simulink model "acc_hardware"  (R2020a)
settings: Solver=VariableStepAuto  StartTime=0.0  StopTime=inf  RelTol=1e-3
libraries: arduinolib x3, arduinosensorlib x1
settings Model: Creator=shesh  LastModifiedBy=shesh

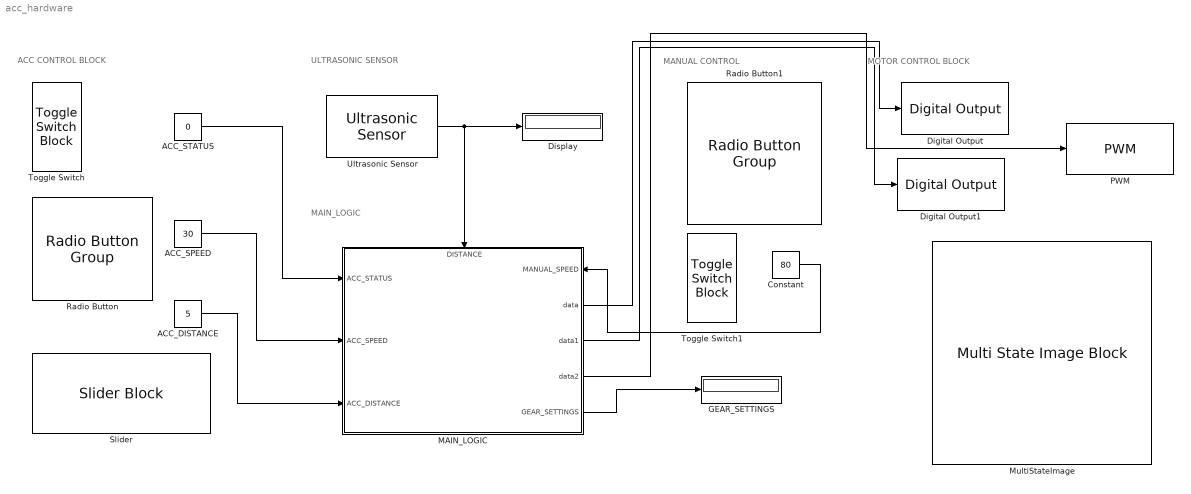
== system acc_hardware ==
  note: MOTOR CONTROL BLOCK
  note: MANUAL CONTROL
  note: MAIN_LOGIC
  note: ULTRASONIC SENSOR
  note: ACC CONTROL BLOCK
  ACC_DISTANCE : Constant  Value=5
  ACC_SPEED : Constant  Value=30
  ACC_STATUS : Constant  Value=0
  Constant : Constant  Value=80
  Digital Output : arduinolib/Digital Output  pinNumber=10  Direction=output  blockPlatform=arduino
  Digital Output1 : arduinolib/Digital Output  pinNumber=9  Direction=output  blockPlatform=arduino
  Display : Display
  GEAR_SETTINGS : Display
  MAIN_LOGIC : Stateflow chart  TreatAsAtomicUnit=on
      settings: PortSchema="{\"entries\":[{\"content\":{\"sides\":[{\"content\":{\"connectorIds\":[\"In3\",\"In4\",\"In5\"]},\"type\":\"ConnectorPlacement.EquallySpacedRectSide\",\"uuid\":\"9577933f-3cd5-4877-b3f1-1cabc5f66bc2\"},{\"content\":{\"connectorIds\":[\"In1\",\"Out1\",\"Out2\",\"Out3\",\"Out4\"],\"side\":\"RIGHT\"},\"type\":\"ConnectorPlacement.EquallySpacedRectSide\",\"uuid\":\"2a6dc85d-fd72-47ef-ac66-14217eaecbf8\"},{\"content\":{\"connectorIds\":[\"In2\"],\"side\":\"TOP\"},\"type\":\"ConnectorPlacement.EquallySpacedRectSide\",\"uuid\":\"38d285f4-ccf6-4804-ae1f-6877806054a5\"}]},\"type\":\"ConnectorPlacement.EquallySpacedConnector\",\"uuid\":\"df4108ed-a8cc-4829-9830-7e09486e0f89\"}],\"packageUris\":[\"http://schema.mathworks.com/mf0/Connector/19700101\"],\"version\":\"1.0\"}"
  MultiStateImage : MultiStateImageBlock
  PWM : arduinolib/PWM  pinNumber=5  frequencyType=Default  desiredFrequency=490.2  achievableFrequency=490.2
  Radio Button : RadioButtonGroup  SelectedLabel=30 KMPH  ButtonGroupName=Group
      settings: Values={{'30 KMPH', '40 KMPH', '50 KMPH', '60 KMPH'}, [30 40 50 60]}
  Radio Button1 : RadioButtonGroup  SelectedLabel=80 KMPH  ButtonGroupName=Group
      settings: Values={{'40 KMPH', '80 KMPH', '120 KMPH', '160 KMPH', 'BREAK'}, [40 80 120 160 0]}
  Slider : SliderBlock  ScaleMin=5  ScaleMax=10  TickInterval=1
  Toggle Switch : ToggleSwitchBlock
      settings: Values={{'Off', 'On'}, [0 1]}
  Toggle Switch1 : ToggleSwitchBlock
      settings: Values={{'Off', 'On'}, [1 0]}
  Ultrasonic Sensor : arduinosensorlib/Ultrasonic Sensor  NumSignalPins=2  TrigPin=4  EchoPin=5  SignalPin=3  SampleTime_=0.1  blockPlatform=ARDUINO
      settings: SourceProductBaseCode=ARDUINO
  wires:
  ACC_STATUS/1 -> MAIN_LOGIC/3(ACC_STATUS)
  ACC_SPEED/1 -> MAIN_LOGIC/4(ACC_SPEED)
  ACC_DISTANCE/1 -> MAIN_LOGIC/5(ACC_DISTANCE)
  MAIN_LOGIC/4(GEAR_SETTINGS) -> GEAR_SETTINGS/1
  Constant/1 -> MAIN_LOGIC/1(MANUAL_SPEED)
  Ultrasonic Sensor/1 -> Display/1, MAIN_LOGIC/2(DISTANCE)
  MAIN_LOGIC/1(data) -> Digital Output/1
  MAIN_LOGIC/2(data1) -> Digital Output1/1
  MAIN_LOGIC/3(data2) -> PWM/1

== stateflow chart acc_hardware/MAIN_LOGIC ==
  state ADAPTIVE_CONTROL_ACTIVE
    entry:
    state ZERO_GEAR_STATE
      entry:
      GEAR_SETTINGS = 0;
    state FRIST_GEAR_STATE
      entry:
      GEAR_SETTINGS = 1;
    state SECOND_GEAR_STATE
      entry:
      GEAR_SETTINGS = 2;
    state BREAKING_STATE
      entry:
      GEAR_SETTINGS = 3;
    (default) -> ADAPTIVE_CONTROL_ACTIVE.ZERO_GEAR_STATE
    ADAPTIVE_CONTROL_ACTIVE.FRIST_GEAR_STATE -> ADAPTIVE_CONTROL_ACTIVE.ZERO_GEAR_STATE : [ACC_SPEED<=40]
    ADAPTIVE_CONTROL_ACTIVE.ZERO_GEAR_STATE -> ADAPTIVE_CONTROL_ACTIVE.FRIST_GEAR_STATE
    ADAPTIVE_CONTROL_ACTIVE.SECOND_GEAR_STATE -> ADAPTIVE_CONTROL_ACTIVE.ZERO_GEAR_STATE : [ACC_SPEED<=40]
    ADAPTIVE_CONTROL_ACTIVE.BREAKING_STATE -> ADAPTIVE_CONTROL_ACTIVE.ZERO_GEAR_STATE : [ACC_SPEED<=40]
  state ADAPTIVE_CONTROL_INACTIVE
    entry:
    state ZERO_GEAR_STATE
      entry:
      GEAR_SETTINGS = 0;
    state FRIST_GEAR_STATE
      entry:
      GEAR_SETTINGS = 1;
    state SECOND_GEAR_STATE
      entry:
      GEAR_SETTINGS = 2;
    state BREAKING_STATE
      entry:
      GEAR_SETTINGS = 3;
    ADAPTIVE_CONTROL_INACTIVE.ZERO_GEAR_STATE -> ADAPTIVE_CONTROL_INACTIVE.FRIST_GEAR_STATE [order 1] : [MANUAL_SPEED == 120]
    ADAPTIVE_CONTROL_INACTIVE.FRIST_GEAR_STATE -> ADAPTIVE_CONTROL_INACTIVE.ZERO_GEAR_STATE [order 3] : [(MANUAL_SPEED == 40) || (MANUAL_SPEED == 80)]
    (default) -> ADAPTIVE_CONTROL_INACTIVE.ZERO_GEAR_STATE
    ADAPTIVE_CONTROL_INACTIVE.ZERO_GEAR_STATE -> ADAPTIVE_CONTROL_INACTIVE.BREAKING_STATE [order 3] : [MANUAL_SPEED == 160]
    ADAPTIVE_CONTROL_INACTIVE.SECOND_GEAR_STATE -> ADAPTIVE_CONTROL_INACTIVE.FRIST_GEAR_STATE [order 1] : [MANUAL_SPEED == 120]
    ADAPTIVE_CONTROL_INACTIVE.SECOND_GEAR_STATE -> ADAPTIVE_CONTROL_INACTIVE.ZERO_GEAR_STATE [order 3] : [(MANUAL_SPEED == 40) || (MANUAL_SPEED == 80)]
    ADAPTIVE_CONTROL_INACTIVE.ZERO_GEAR_STATE -> ADAPTIVE_CONTROL_INACTIVE.SECOND_GEAR_STATE [order 2] : [MANUAL_SPEED == 160]
    ADAPTIVE_CONTROL_INACTIVE.BREAKING_STATE -> ADAPTIVE_CONTROL_INACTIVE.ZERO_GEAR_STATE [order 3] : [(MANUAL_SPEED == 40) || (MANUAL_SPEED == 80)]
    ADAPTIVE_CONTROL_INACTIVE.FRIST_GEAR_STATE -> ADAPTIVE_CONTROL_INACTIVE.SECOND_GEAR_STATE [order 1] : [MANUAL_SPEED == 160]
    ADAPTIVE_CONTROL_INACTIVE.BREAKING_STATE -> ADAPTIVE_CONTROL_INACTIVE.FRIST_GEAR_STATE [order 1] : [MANUAL_SPEED == 120]
    ADAPTIVE_CONTROL_INACTIVE.FRIST_GEAR_STATE -> ADAPTIVE_CONTROL_INACTIVE.BREAKING_STATE [order 2] : [MANUAL_SPEED == 160]
    ADAPTIVE_CONTROL_INACTIVE.SECOND_GEAR_STATE -> ADAPTIVE_CONTROL_INACTIVE.BREAKING_STATE [order 2] : [MANUAL_SPEED == 160]
    ADAPTIVE_CONTROL_INACTIVE.BREAKING_STATE -> ADAPTIVE_CONTROL_INACTIVE.SECOND_GEAR_STATE [order 2] : [MANUAL_SPEED == 160]
  (default) -> ADAPTIVE_CONTROL_ACTIVE
  ADAPTIVE_CONTROL_ACTIVE -> ADAPTIVE_CONTROL_INACTIVE : [ACC_STATUS == 0]
  ADAPTIVE_CONTROL_INACTIVE -> ADAPTIVE_CONTROL_ACTIVE : [ACC_STATUS == 1]
  data: data output; data1 output; data2 output; MANUAL_SPEED input; DISTANCE input; ACC_STATUS input; ACC_SPEED input; ACC_DISTANCE input; GEAR_SETTINGS output
